simulink model "Driver_TS9"  (R2014b)
settings: Solver=ode45  StartTime=0.0  StopTime=15  RelTol=1e-3
InitFcn:
  | clear
  | clc
  | load('data');
libraries: Solver_SF x1
settings Model: Creator=zhaolingfeng  LastModifiedBy=zhaolingfeng

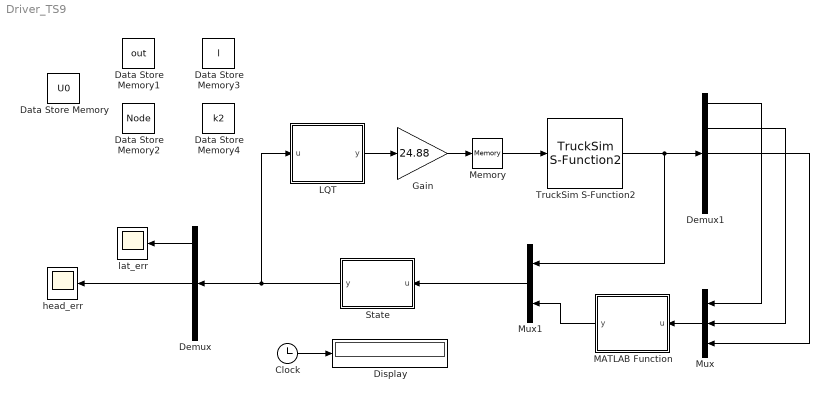
== system Driver_TS9 ==
  Clock : Clock
  Data Store Memory : DataStoreMemory  DataStoreName=U0  ReadBeforeWriteMsg=warning  WriteAfterWriteMsg=warning  WriteAfterReadMsg=warning  OutDataTypeStr=double
  Data Store Memory1 : DataStoreMemory  DataStoreName=out  ReadBeforeWriteMsg=warning  WriteAfterWriteMsg=warning  WriteAfterReadMsg=warning  InitialValue=out  OutDataTypeStr=double
  Data Store Memory2 : DataStoreMemory  DataStoreName=Node  ReadBeforeWriteMsg=warning  WriteAfterWriteMsg=warning  WriteAfterReadMsg=warning  InitialValue=Node  OutDataTypeStr=double
  Data Store Memory3 : DataStoreMemory  DataStoreName=l  ReadBeforeWriteMsg=warning  WriteAfterWriteMsg=warning  WriteAfterReadMsg=warning  InitialValue=l  OutDataTypeStr=double
  Data Store Memory4 : DataStoreMemory  DataStoreName=k2  ReadBeforeWriteMsg=warning  WriteAfterWriteMsg=warning  WriteAfterReadMsg=warning  InitialValue=k2  OutDataTypeStr=double
  Demux : Demux  Outputs=[1 1 3]
  Demux1 : Demux  Outputs=5
  Display : Display
      settings: Format=bank  Decimation=100
  Gain : Gain  Gain=24.88
  LQT : MATLAB Function  TreatAsAtomicUnit=on  SystemSampleTime=0.2
  MATLAB Function : MATLAB Function  TreatAsAtomicUnit=on  SystemSampleTime=0.2
  Memory : Memory
  Mux : Mux  Inputs=3
  Mux1 : Mux  Inputs=2
  State : MATLAB Function  TreatAsAtomicUnit=on  SystemSampleTime=0.2
  TruckSim S-Function2 : Solver_SF/TruckSim S-Function2  Priority=1  VehicleCode=f_s_s__ss  SIMFILE=simfile.sim
      settings: AttributesFormatString=Vehicle Code: %<VehicleCode>
  head_err : Scope
  lat_err : Scope
  wires:
  TruckSim S-Function2/1 -> Mux1/1, Demux1/1
  Clock/1 -> Display/1
  Demux1/3 -> Mux/3
  Demux1/1 -> Mux/1
  Mux/1 -> MATLAB Function/1(u)
  Demux1/2 -> Mux/2
  MATLAB Function/1(y) -> Mux1/2
  State/1(y) -> Demux/1, LQT/1(u)
  LQT/1(y) -> Gain/1
  Mux1/1 -> State/1(u)
  Demux/1 -> lat_err/1
  Demux/2 -> head_err/1
  Gain/1 -> Memory/1
  Memory/1 -> TruckSim S-Function2/1

== matlab function Driver_TS9/State ==
  data: u input; y output
function y = fcn(u)
%#codegen
X = u(1);
Y = u(2);
Yaw = u(3)/180*pi;
Hangle = u(4)/180*pi;
Vx = u(5)*1000/3600;

% 基准为后轴中心
l2 = 6.7; % 拖车轴距
X = X - l2*cos(Yaw);
Y = Y - l2*sin(Yaw);

Xt = u(6);
Yt = u(7);
theta = u(8);
target_s = u(9);

lat_err = - (X-Xt)*sin(theta) + (Y-Yt)*cos(theta);
yaw_err = Yaw - theta;

y = [lat_err yaw_err Hangle Vx target_s]';

== matlab function Driver_TS9/MATLAB Function ==
  data: u input; y output; out data_store_memory; Node data_store_memory; k2 data_store_memory; l data_store_memory
function y = fcn(u)
%#codegen
global out Node k2 l;
X = u(1);
Y = u(2);
Yaw = u(3)/180*pi;

% 基准为后轴中心
l2 = 6.7; % 拖车轴距
X = X - l2*cos(Yaw);
Y = Y - l2*sin(Yaw);

min_idx1 = 0; min_idx2 = 0;
min_d1 = 50; min_d2 = 50;
for i = 1:length(out(:,1))
    dist = sqrt((out(i,1)-X)^2 + (out(i,2)-Y)^2);
    if dist < min_d2
        if dist < min_d1
            min_d2 = min_d1; min_idx2 = min_idx1;
            min_d1 = dist; min_idx1 = i;
        else
            min_d2 = dist; min_idx2 = i;
        end
    end
end

% 求解最近点s
dist = ([X Y] - [Node(1,3) Node(2,3)]) * [0 1]'; % 延长线
if dist > 0
    target_s = Node(3,3) + dist;
else
    if min_idx1 > min_idx2
        tmp_idx = min_idx1;
        min_idx1 = min_idx2;
        min_idx2 = tmp_idx;
    end
    v0 = [out(min_idx1,1) out(min_idx1,2)] - [out(min_idx2,1) out(min_idx2,2)];
    va = [X Y] - [out(min_idx1,1) out(min_idx1,2)];
    % 按照投影长度插值求最近点s
    target_s = out(min_idx1,3) + (out(min_idx2,3)-out(min_idx1,3))*abs(va*v0'/norm(v0)^2);
end

% 求解目标位置&航向
if target_s <= Node(3,1)
    [Xt, Yt, theta, ~] = seg1(out(min_idx1,1), out(min_idx1,2), out(min_idx1,3), (out(min_idx1,3)+target_s)/2, target_s, k2, l);
elseif target_s <= Node(3,2)
    [Xt, Yt, theta, ~] = seg2(X, Y, Node, k2, l);
elseif target_s <= Node(3,3)
    [Xt, Yt, theta, ~] = seg3(out(min_idx1,1), out(min_idx1,2), out(min_idx1,3)-Node(3,2), (out(min_idx1,3)+target_s)/2-Node(3,2), target_s-Node(3,2), k2, l);
else
    Xt = Node(1,3);
    Yt = Node(2,3) + dist;
    theta = pi/2;
end

y = [Xt Yt theta target_s]';

== matlab function Driver_TS9/LQT ==
  data: u input; y output; U0 data_store_memory; Node data_store_memory; k2 data_store_memory; l data_store_memory
function y = fcn(u)
%#codegen
lat_err = u(1);
yaw_err = u(2);
Hangle = u(3);
Vx = u(4);
target_s = u(5);

l1 = 4.0; % 牵引车轴距
l2 = 6.7; % 拖车轴距
lh = 1.0; % 挂钩位置

T = 0.2; % 控制频率
Tsim = 8; % 预测时域

% 提取道路信息
global Node k2 l;
kc = k2*l^2/2;
ss = target_s;
curv = zeros(2,Tsim); Yt = zeros(3,Tsim);
for i = 1:Tsim
    if ss <= Node(3,1)
        % 第一段
        if ss <= l/2
            curv(:,i) = [k2*ss^2 2*k2*ss]'; % 曲率 曲率变化率
        else
            curv(:,i) = [-k2*ss^2+2*k2*l*ss-k2*l^2/2 -2*k2*ss+2*k2*l]';
        end
    elseif ss <= Node(3,2)
        curv(:,i) = [kc 0]';
    elseif ss <= Node(3,3)
        skp = ss - Node(3,2);
        if skp <= l/2
            curv(:,i) = [-k2*skp^2+kc -2*k2*skp]';
        else
            curv(:,i) = [k2*skp^2-2*k2*l*skp+k2*l^2/2+kc 2*k2*skp-2*k2*l]';
        end
    else
        curv(:,i) = [0 0]';
    end
    Yt(:,i) = [0 0 Vx*curv(1,i)]';
    ss = ss + Vx*T;
end

% 初始状态
x_0 = [lat_err;
    yaw_err];
global U0;
x_0 = [x_0; U0]; %上一时刻的控制量

Q = diag([1.0 1.5 7.0]);
R = 0.05;

% 连续时间模型
% 状态转移矩阵
A = [0    Vx;
    0    0];

% 控制矩阵
B = [0;
    1];

% 扰动矩阵
C = [0;
    -1];

% 观测矩阵
D = eye(2);

%离散化
A_d = inv(eye(length(A)) - T*A/2) * (eye(length(A)) + T*A/2); % 双线性变换
% A_d = eye(length(A)) + T*A;
B_d = B*T;
C_d = C*T;

%变为增量
A_d = [A_d      B_d;
    zeros(1,2) eye(1)];
B_d = [B_d; eye(1)];
C_d = [C_d; 0];
D = [D zeros(2,1);
    0 0 1];

% 递推求解增益 K & Kv
K = zeros(Tsim-1,3);
Kv = zeros(Tsim-1,3);
S = zeros(3,3,Tsim);
S(:,:,Tsim) = D'*Q*D;
v = zeros(3,Tsim);
v(:,Tsim) = D'*Q*Yt(:,end);
for i = Tsim-1:-1:1
    Kv(i,:) = ( R + B_d'*S(:,:,i+1)*B_d ) \ B_d';
    K(i,:) = Kv(i,:) * S(:,:,i+1);
    S(:,:,i) = A_d'*(S(:,:,i+1) - S(:,:,i+1)*B_d*K(i,:))*A_d + D'*Q*D;
    dd = C_d*Vx*curv(1,i); % 扰动项
    v(:,i) = (A_d - B_d*K(i,:)*A_d)'*v(:,i+1) - A_d'*S(:,:,i+1)*(eye(3)-B_d*K(i,:))*dd + D'*Q*Yt(:,i);
end

% 求解控制量
dd = C_d*Vx*curv(1,1);
ufb = -K(1,:)*(A_d*x_0+dd) + Kv(1,:)*v(:,2) + x_0(end);
U0 = ufb;

tmp_angle = atan(ufb*l2/Vx);
thetaf = atan( tan(tmp_angle + Hangle)*l1/lh ); % 转换为前轮转角

y = thetaf*180/pi;
